simulink subsystem "MEKF_verify"  (R2024a)
settings: Solver=VariableStepAuto  StartTime=0.0  StopTime=10.0  RelTol=1e-3
libraries: aerolibutil x2
settings Model: Creator=joshu  LastModifiedBy=joshu

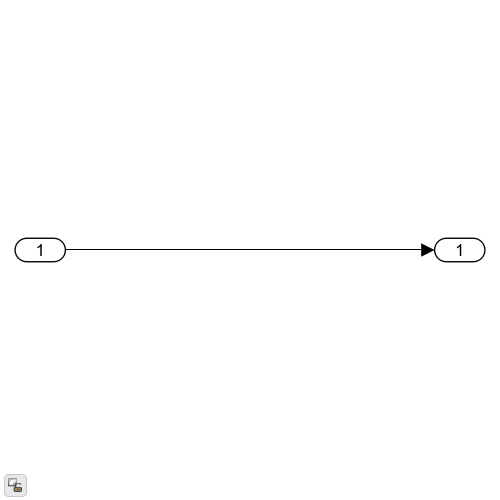
[thumbnail: Simulink's stored preview of the top-level diagram]
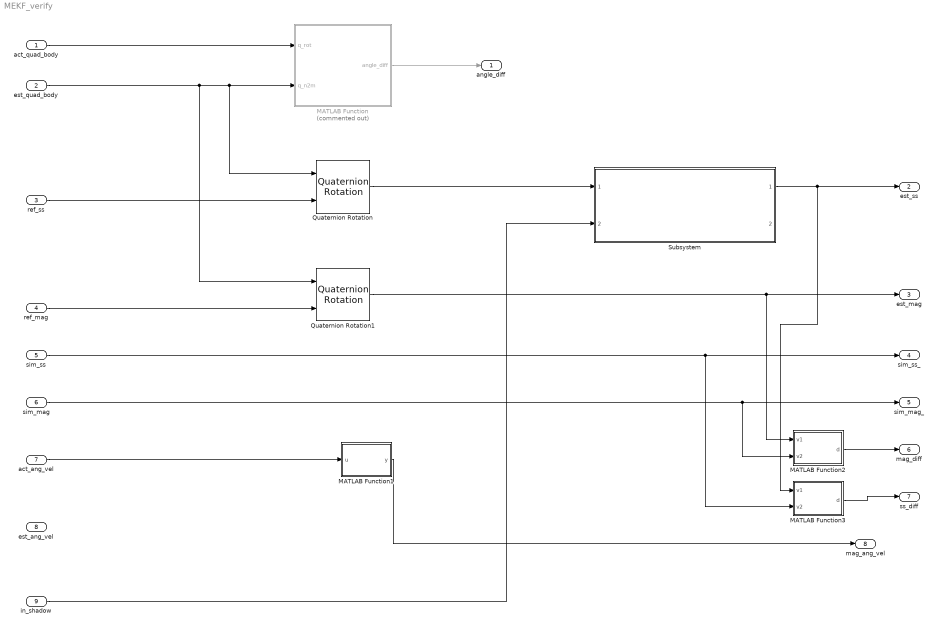
== system MEKF_verify ==
  act_quad_body : Inport
  est_quad_body : Inport  Port=2
  ref_ss : Inport  Port=3
  ref_mag : Inport  Port=4
  sim_ss : Inport  Port=5
  sim_mag : Inport  Port=6
  act_ang_vel : Inport  Port=7
  est_ang_vel : Inport  Port=8
  in_shadow : Inport  Port=9
  MATLAB Function : MATLAB Function  Commented=on  TreatAsAtomicUnit=on
  MATLAB Function1 : MATLAB Function  TreatAsAtomicUnit=on
  MATLAB Function2 : MATLAB Function  TreatAsAtomicUnit=on
  MATLAB Function3 : MATLAB Function  TreatAsAtomicUnit=on
  Quaternion Rotation : aerolibutil/Quaternion Rotation
  Quaternion Rotation1 : aerolibutil/Quaternion Rotation
  Subsystem : Subsystem  ReferencedSubsystem=sun_sensor_model
  angle_diff : Outport
  est_ss : Outport  Port=2
  est_mag : Outport  Port=3
  sim_ss_ : Outport  Port=4
  sim_mag_ : Outport  Port=5
  mag_diff : Outport  Port=6
  ss_diff : Outport  Port=7
  mag_ang_vel : Outport  Port=8
  wires:
  act_quad_body/1 -> MATLAB Function/1(q_rot)
  est_quad_body/1 -> MATLAB Function/2(q_n2m), Quaternion Rotation/1, Quaternion Rotation1/1
  act_ang_vel/1 -> MATLAB Function1/1(u)
  MATLAB Function/1(angle_diff) -> angle_diff/1
  ref_ss/1 -> Quaternion Rotation/2
  ref_mag/1 -> Quaternion Rotation1/2
  in_shadow/1 -> Subsystem/2
  Quaternion Rotation/1 -> Subsystem/1
  Quaternion Rotation1/1 -> est_mag/1, MATLAB Function2/1(v1)
  sim_ss/1 -> sim_ss_/1, MATLAB Function3/2(v2)
  sim_mag/1 -> sim_mag_/1, MATLAB Function2/2(v2)
  Subsystem/1 -> est_ss/1, MATLAB Function3/1(v1)
  MATLAB Function1/1(y) -> mag_ang_vel/1
  MATLAB Function2/1(d) -> mag_diff/1
  MATLAB Function3/1(d) -> ss_diff/1

== matlab function MEKF_verify/MATLAB Function ==
  data: q_rot input; angle_diff output; q_n2m input
function angle_diff = fcn(q_rot,q_n2m)

angle_diff = quad_dangle(q_rot,q_n2m);

== matlab function MEKF_verify/MATLAB Function2 ==
  data: v1 input; d output; v2 input
function d = fcn(v1,v2)
d = vector_dangle(v1,v2);

== matlab function MEKF_verify/MATLAB Function3 ==
  data: v1 input; d output; v2 input
function d = fcn(v1,v2)
d = sum(abs(acosd(v1) - acosd(v2)));

== matlab function MEKF_verify/MATLAB Function1 ==
  data: u input; y output
function y = fcn(u)

y = norm(u);

%if y > 10
%    disp(y)
%    disp(u)
%    error("Satelite is tumbelling")
end
